simulink model "notchFilterSimulink"  (R2018b)
settings: Solver=VariableStepAuto  StartTime=0.0  StopTime=100  RelTol=1e-3
undefined symbols (not defined in the file): p11, p12, p13, p21, p22, p23, Te
libraries: simulink x1
settings Model: Creator=Asus  LastModifiedBy=Asus

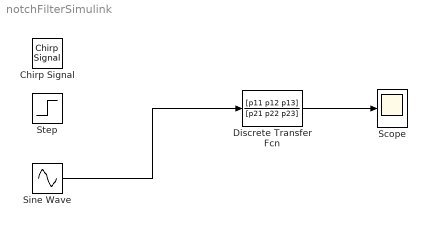
== system notchFilterSimulink ==
  Chirp Signal : simulink/Sources/Chirp Signal  f1=1  T=10  f2=500
  Discrete Transfer Fcn : DiscreteTransferFcn  Numerator=[p11 p12 p13]  Denominator=[p21 p22 p23]  SampleTime=Te
  Scope : Scope
  Sine Wave : Sin  Amplitude=51  Frequency=50  SampleTime=Te
  Step : Step  Time=0  SampleTime=Te
  wires:
  Discrete Transfer Fcn/1 -> Scope/1
  Sine Wave/1 -> Discrete Transfer Fcn/1
